simulink model "sl_quadrotorDynamics"  (R2019b)
settings: Solver=VariableStepAuto  StartTime=0.0  StopTime=50  MaxStep=0.1  RelTol=1e-3  EnableMultiTasking=on
InitFcn:
  | % load parameters of the default quadrotor
  | disp('Quadrotor parameters loaded by InitFcn')
  | mdl_quadrotor
values from neighbouring files (symbols this model uses):
  pp_cont =     [sim_parameters.mat]
undefined symbols (not defined in the file or in its folder): quad
libraries: roblocks x1, simulink x1
settings Model: Creator=corkep
settings DataIOCC: LimitDataPoints=on  SaveFormat=Array  ReturnWorkspaceOutputs=off
settings OptimizationCC: BlockReduction=off  BooleanDataType=off  LifeSpan=inf
settings DebuggingCC: SaveWithParameterizedLinksMsg=none  UnderspecifiedInitializationDetection=Classic  MergeDetectMultiDrivingBlocksExec=none  SignalResolutionControl=TryResolveAllWithWarning  SFUnexpectedBacktrackingDiag=warning  SFNoUnconditionalDefaultTransitionDiag=warning  SFExecutionAtInitializationDiag=none  ArithmeticOperatorsInVariantConditions=warning
settings HardwareCC: ProdBitPerPointer=32  ProdBitPerSizeT=32  ProdBitPerPtrDiffT=32  ProdLargestAtomicFloat=None  ProdIntDivRoundTo=Undefined  ProdEndianess=Unspecified  ProdWordSize=32  ProdHWDeviceType=32-bit Generic  TargetUnknown=on
settings ModelReferenceCC: PropagateSignalLabelsOutOfModel=off
settings SFSimCC: SimUseLocalCustomCode=off  CustomCodeUndefinedFunction=UseInterfaceOnly
settings RTWCC: RTWUseLocalCustomCode=off
settings CodeAppCC: StateflowObjectComments=on
settings GRTTargetCC: TargetLangStandard=C89/C90 (ANSI)  GeneratePreprocessorConditionals=Disable all
settings ConfigComp: CovMetricSettings=dw  CovHtmlReporting=on  CovSaveCumulativeToWorkspaceVar=on  CovSaveSingleToWorkspaceVar=on  CovExternalEMLEnable=off  CovSFcnEnable=off

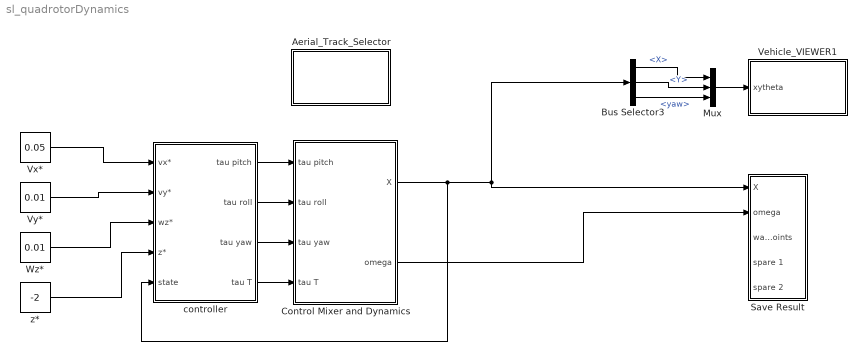
== system sl_quadrotorDynamics ==
  " Save Result" : Subsystem
  Aerial_Track_Selector : Subsystem  mask{the_XL_filename=aerial_robot_waypoints.xlsx, the_racetrack_str=RECT_TRI, the_look_ahead_dist=0.3, the_des_lin_vel=0.1, the_max_ang_vel_deg_sec=60}
      mask prompts: the_XL_filename "EXCEL file (eg: bh.xlsx)"; the_racetrack_str "Racetrack type"; the_look_ahead_dist "Look ahead distance (m)"; the_des_lin_vel "Desired Linear Velocity (m/sec)"; the_max_ang_vel_deg_sec "Max Angular Velocity (deg/sec)"
      mask init:
      | %fprintf('\n ... <%s> and <%s>',the_XL_filename, the_racetrack_str);
      | 
      | A_MASK_OBJ  = Simulink.Mask.get(gcb);
      | A_IMAGE_OBJ = A_MASK_OBJ.getDialogControl('the_track_pic_param');
      | A_IMAGE_OBJ.FilePath = [the_racetrack_str,'.png'];
      | 
      | %--------------------------------------------------------------
      | THE_FILE  = the_XL_filename; 
      | THE_SHEET = the_racetrack_str;
      | my_path_data_T = readtable(THE_FILE, 'Sheet', THE_SHEET);
      | 
      | assignin('base', 'my_path_data_T', my_path_data_T );
      | evalin(  'base', 'pp_cont.Waypoints = [my_path_data_T.X,  my_path_data_T.Y ];' );
      | evalin('base', 'close all');
      | %--------------------------------------------------------------
      | evalin('base', ['pp_cont.LookaheadDistance=',num2str(the_look_ahead_dist),';']);
      | evalin('base', ['pp_cont.DesiredLinearVelocity=',num2str(the_des_lin_vel),';']);
      | evalin('base', ['pp_cont.MaxAngularVelocity=',num2str(the_max_ang_vel_deg_sec*pi/180),';']);
      | %pp_cont.LookaheadDistance     = 0.2;        % m 
      | %pp_cont.DesiredLinearVelocity = 0.1;        % m/s
      | %pp_cont.MaxAngularVelocity    = 60*pi/180;  %radians/second
      mask TypeOptions the_racetrack_str: SPANNER | RECT_TRI | MEDIUM_S_HOME | SMALL_S_HOME | SQUARE | CIRCLE_HOME | L_AND_R_TURNS
      mask DialogControl DescGroupVar Prompt: m_RaceTrack_Selector
      mask DialogControl DescTextVar Prompt: Select the racetrack for your Differential Drive Robot (DDR).  And specify the parameters for your Pure Pursuit controller.
      mask DialogControl Container10 Prompt: RaceTrack
      mask DialogControl Container5 Prompt: PurePursuit
      mask DialogControl Control4 Prompt: If you want some DEFAULT values then click on the button below
      mask DialogControl the_set_def_PP_values Prompt: Set Default values
      mask DialogControl the_set_def_PP_values Callback:
      | set_param(gcb,'the_look_ahead_dist','0.2');
      | set_param(gcb,'the_des_lin_vel','0.1');
      | set_param(gcb,'the_max_ang_vel_deg_sec','60');
      | fprintf('\n *** applied DEFAULT values to PP params ***');
      mask DialogControl Control2 Prompt: As a general rule, the lookahead distance should be larger than the desired linear velocity for a smooth path. The robot might cut corners when the lookahead distance is large. In contrast, a small lookahead distance can result in an unstable path following behavior.
      mask Display: fprintf('%s',the_racetrack_str)
  Bus Selector3 : BusSelector  OutputSignals=X,Y,yaw
  Control Mixer and Dynamics : Subsystem
  Mux : Mux  Inputs=3
  Vehicle_VIEWER1 : Subsystem  mask{wp_mat=pp_cont.Waypoints, veh_ID_num=1, veh_init_xytheta=[0 0 0], Ts=0.1}
      mask prompts: wp_mat "Waypoint matrix for arena [x_col, y_col, z_col, angle_col] (m, deg)"; veh_ID_num "Vehicle ID number"; veh_init_xytheta "Initial pose [x,y, psi]"; Ts "Sample time for updating animation (secs)"
      mask TypeOptions veh_ID_num: 1 | 2 | 3 | 4
      mask DialogControl Control2 Prompt: Animate simulation of Robot
      mask Display: fprintf('veh_ID=%d',veh_ID_num);
  Vx* : Constant  Value=0.05
  Vy* : Constant  Value=0.01
  Wz* : Constant  Value=0.01
  controller : Subsystem
  z* : Constant  Value=-2
  wires:
  Control Mixer and Dynamics/2(omega) -> " Save Result"/2(omega)
  Control Mixer and Dynamics/1(X) -> controller/5(state), Bus Selector3/1, " Save Result"/1(X)
  Bus Selector3/1 -> Mux/1  "<X>"
  Mux/1 -> Vehicle_VIEWER1/1(xytheta)
  Bus Selector3/2 -> Mux/2  "<Y>"
  Bus Selector3/3 -> Mux/3  "<yaw>"
  controller/3(tau yaw) -> Control Mixer and Dynamics/3(tau yaw)
  controller/4(tau T) -> Control Mixer and Dynamics/4(tau T)
  Wz*/1 -> controller/3(wz*)
  z*/1 -> controller/4(z*)
  controller/1(tau pitch) -> Control Mixer and Dynamics/1(tau pitch)
  controller/2(tau roll) -> Control Mixer and Dynamics/2(tau roll)
  Vx*/1 -> controller/1(vx*)
  Vy*/1 -> controller/2(vy*)

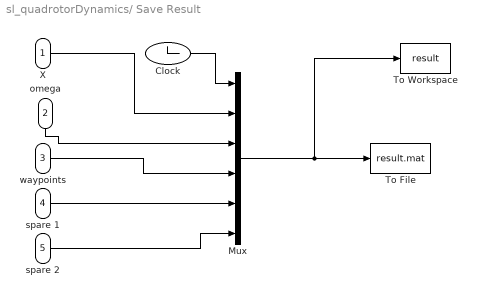
== system sl_quadrotorDynamics/ Save Result ==
  X : Inport
  omega : Inport  Port=2
  waypoints : Inport  Port=3
  spare 1 : Inport  Port=4
  spare 2 : Inport  Port=5
  Clock : Clock
  Mux : Mux  Inputs=6
  To File : ToFile  Filename=result.mat  MatrixName=result  SaveFormat=Timeseries
  To Workspace : ToWorkspace  VariableName=result  SampleTime=-1
  wires:
  Clock/1 -> Mux/1
  omega/1 -> Mux/3
  Mux/1 -> To Workspace/1, To File/1
  X/1 -> Mux/2
  spare 1/1 -> Mux/5
  spare 2/1 -> Mux/6
  waypoints/1 -> Mux/4

== system sl_quadrotorDynamics/Aerial_Track_Selector ==

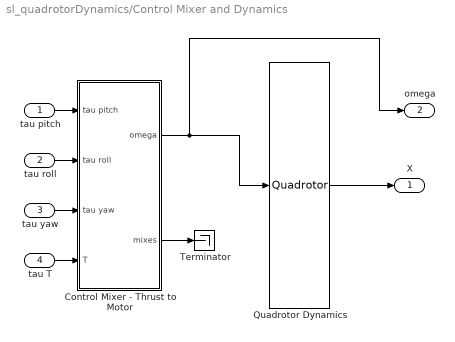
== system sl_quadrotorDynamics/Control Mixer and Dynamics ==
  tau pitch : Inport
  tau roll : Inport  Port=2
  tau yaw : Inport  Port=3
  tau T : Inport  Port=4
  Control Mixer - Thrust to Motor : Subsystem
  Quadrotor Dynamics : roblocks/Dynamics/Quadrotor  quad=quad
      link override Dynamics: FunctionName=nrotor_dynamics
  Terminator : Terminator
  X : Outport  VectorParamsAs1DForOutWhenUnconnected=off
  omega : Outport  Port=2  VectorParamsAs1DForOutWhenUnconnected=off
  wires:
  Quadrotor Dynamics/1 -> X/1
  Control Mixer - Thrust to Motor/2(mixes) -> Terminator/1
  tau pitch/1 -> Control Mixer - Thrust to Motor/1(tau pitch)
  tau roll/1 -> Control Mixer - Thrust to Motor/2(tau roll)
  tau yaw/1 -> Control Mixer - Thrust to Motor/3(tau yaw)
  tau T/1 -> Control Mixer - Thrust to Motor/4(T)
  Control Mixer - Thrust to Motor/1(omega) -> Quadrotor Dynamics/1, omega/1

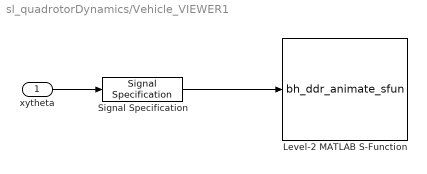
== system sl_quadrotorDynamics/Vehicle_VIEWER1 ==
  xytheta : Inport
  Level-2 MATLAB S-Function : M-S-Function  FunctionName=bh_ddr_animate_sfun  Parameters=Ts, wp_mat, veh_ID_num, veh_init_xytheta
  Signal Specification : SignalSpecification  Dimensions=3
  wires:
  xytheta/1 -> Signal Specification/1
  Signal Specification/1 -> Level-2 MATLAB S-Function/1

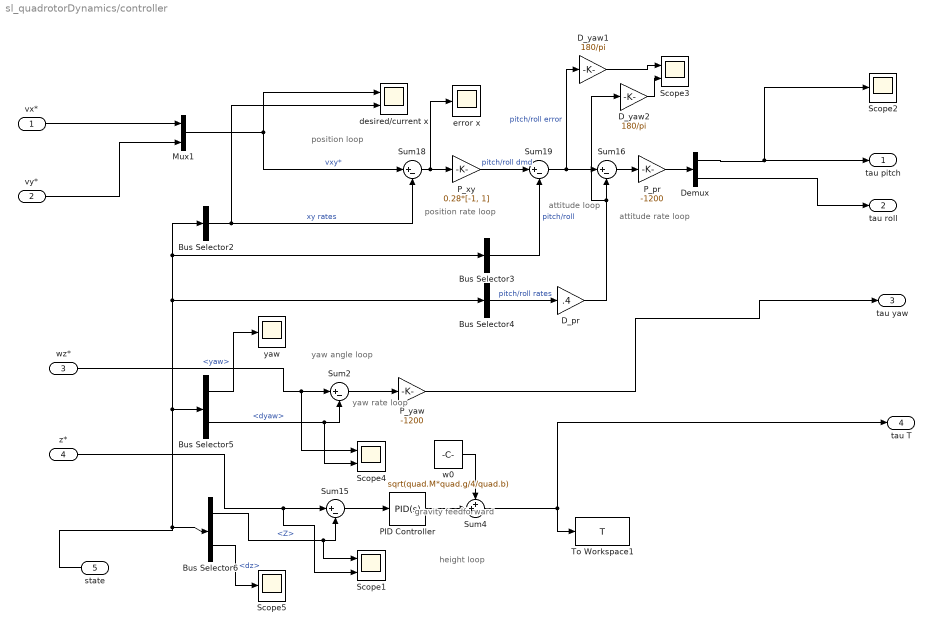
== system sl_quadrotorDynamics/controller ==
  note: gravity feedforward
  note: attitude rate
      | loop
  note: attitude
      | loop
  note: position rate
      | loop
  note: position
      | loop
  note: yaw rate
      | loop
  note: yaw angle
      | loop
  note: height
      | loop
  vx* : Inport
  vy* : Inport  Port=2
  wz* : Inport  Port=3
  z* : Inport  Port=4
  state : Inport  Port=5
  Bus Selector2 : BusSelector  OutputSignals=dx,dy  OutputAsBus=on
  Bus Selector3 : BusSelector  OutputSignals=pitch,roll  OutputAsBus=on
  Bus Selector4 : BusSelector  OutputSignals=dpitch,droll  OutputAsBus=on
  Bus Selector5 : BusSelector  OutputSignals=yaw,dyaw
  Bus Selector6 : BusSelector  OutputSignals=Z,dz
  D_pr : Gain  Gain=.4
  D_yaw1 : Gain  Gain=180/pi
  D_yaw2 : Gain  Gain=180/pi
  Demux : Demux  Outputs=2
  Mux1 : Mux  Inputs=2
  PID Controller : simulink/Continuous/PID Controller  Controller=PID  Form=Parallel  TimeDomain=Continuous-time  SampleTime=-1  IntegratorMethod=Forward Euler  FilterMethod=Forward Euler  ControllerParametersSource=internal  P=-8.79853091186098  I=-0.449865753789399  D=-42.04549910981  UseFilter=on  N=5.45397025421619  TunerSelectOption=Transfer Function Based (PID Tuner App)  InitialConditionSource=internal  InitialConditionForIntegrator=0  InitialConditionForFilter=0  DifferentiatorICPrevScaledInput=0  ExternalReset=none  TrackingMode=off  Kt=1  LimitOutput=off  UpperSaturationLimit=inf  LowerSaturationLimit=-inf  LinearizeAsGain=on  AntiWindupMode=none  Kb=1  POutMin=[]  POutMax=[]  IOutMin=[]  IOutMax=[]  DOutMin=[]  DOutMax=[]  NOutMin=[]  NOutMax=[]  SumOutMin=[]  SumOutMax=[]  SaturationOutMin=[]  SaturationOutMax=[]  PParamMin=[]  PParamMax=[]  IParamMin=[]  IParamMax=[]  DParamMin=[]  DParamMax=[]  NParamMin=[]  NParamMax=[]  KbParamMin=[]  KbParamMax=[]  KtParamMin=[]  KtParamMax=[]  KbOutMin=[]  KbOutMax=[]  KtOutMin=[]  KtOutMax=[]  IntegratorOutMin=[]  IntegratorOutMax=[]  FilterOutMin=[]  FilterOutMax=[]  SumI1OutMin=[]  SumI1OutMax=[]  SumI2OutMin=[]  SumI2OutMax=[]  SumI3OutMin=[]  SumI3OutMax=[]  SumI4OutMin=[]  SumI4OutMax=[]  SumDOutMin=[]  SumDOutMax=[]  DifferentiatorOutMin=[]  DifferentiatorOutMax=[]  FilterDiffOutCoefMin=[]  FilterDiffOutCoefMax=[]  ReciprocalOutMin=[]  ReciprocalOutMax=[]  SumDenOutMin=[]  SumDenOutMax=[]  SumNumOutMin=[]  SumNumOutMax=[]  DivideOutMin=[]  DivideOutMax=[]  IntegratorContinuousStateAttributes=''  IntegratorStateMustResolveToSignalObject=off  IntegratorRTWStateStorageClass=Auto  FilterContinuousStateAttributes=''  FilterStateMustResolveToSignalObject=off  FilterRTWStateStorageClass=Auto  ParallelPVariant=InternalParameters  IdealPVariant=Disabled  IVariant=InternalParameters  DVariant=InternalParameters  IntegratorVariant=Continuous  SatVariant=Disabled  AWVariant=Passthrough  PCopyVariant=Disabled  TRVariant=Disabled  FdbkBlocksVariant=Forward  IdealPFdbkVariant=Disabled  SatFdbkVariant=Disabled  DerivativeFilterVariant=ContFilter  NVariant=InternalParameters  NCopyVariant=Disabled  FilterICVariant=InternalICsFilter  IntegratorICVariant=InternalICs  ExternalResetVariant=Disabled  TRSumVariant=Passthrough  SumFdbkVariant=Disabled  SumVariant=Sum_PID
  P_pr : Gain  Gain=-1200
  P_xy : Gain  Gain=0.28*[-1, 1]
  P_yaw : Gain  Gain=-1200
  Scope1 : Scope  NumInputPorts=2
  Scope2 : Scope
  Scope3 : Scope  NumInputPorts=2
  Scope4 : Scope  NumInputPorts=2
  Scope5 : Scope
  Sum{2,15..16,18..19} (5 alike) : Sum  Inputs=|+-
  Sum4 : Sum  Inputs=++|
  To Workspace1 : ToWorkspace  VariableName=T  SampleTime=-1
  desired/current x : Scope  NumInputPorts=2
  error x : Scope
  w0 : Constant  Value=sqrt(quad.M*quad.g/4/quad.b)  SampleTime=0
  yaw : Scope
  tau pitch : Outport
  tau roll : Outport  Port=2
  tau yaw : Outport  Port=3
  tau T : Outport  Port=4
  wires:
  PID Controller/1 -> Sum4/2
  D_yaw1/1 -> Scope3/1
  Bus Selector2/1 -> Sum18/2, desired/current x/2  "xy rates"
  vy*/1 -> Mux1/2
  P_yaw/1 -> tau yaw/1
  Demux/1 -> tau pitch/1, Scope2/1
  P_pr/1 -> Demux/1
  w0/1 -> Sum4/1
  Sum18/1 -> error x/1, P_xy/1
  Sum15/1 -> PID Controller/1
  D_pr/1 -> D_yaw2/1, Sum16/2
  Sum19/1 -> D_yaw1/1, Sum16/1  "pitch/roll error"
  Mux1/1 -> Sum18/1, desired/current x/1  "vxy*"
  Bus Selector5/2 -> Sum2/2, Scope4/2  "<dyaw>"
  Sum4/1 -> To Workspace1/1, tau T/1
  Demux/2 -> tau roll/1
  wz*/1 -> Scope4/1, Sum2/1
  Bus Selector3/1 -> Sum19/2  "pitch/roll"
  Sum2/1 -> P_yaw/1
  Sum16/1 -> P_pr/1
  state/1 -> Bus Selector4/1, Bus Selector3/1, Bus Selector2/1, Bus Selector5/1, Bus Selector6/1
  P_xy/1 -> Sum19/1  "pitch/roll dmd"
  Bus Selector4/1 -> D_pr/1  "pitch/roll rates"
  vx*/1 -> Mux1/1
  z*/1 -> Scope1/2, Sum15/1
  D_yaw2/1 -> Scope3/2
  Bus Selector6/1 -> Scope1/1, Sum15/2  "<Z>"
  Bus Selector6/2 -> Scope5/1  "<dz>"
  Bus Selector5/1 -> yaw/1  "<yaw>"

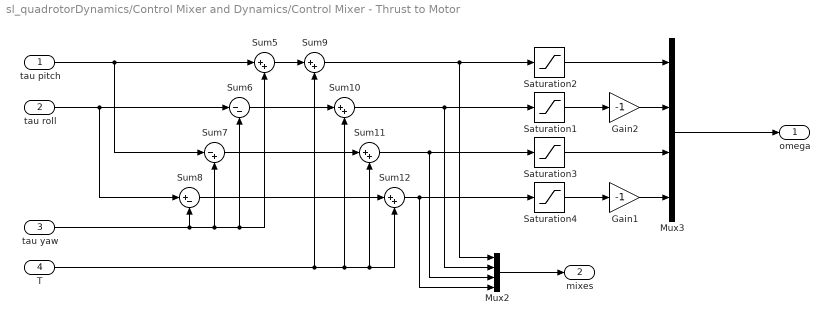
== system sl_quadrotorDynamics/Control Mixer and Dynamics/Control Mixer - Thrust to Motor ==
  tau pitch : Inport
  tau roll : Inport  Port=2
  tau yaw : Inport  Port=3
  T : Inport  Port=4
  Gain1 : Gain  Gain=-1
  Gain2 : Gain  Gain=-1
  Mux2 : Mux
  Mux3 : Mux
  Saturation{1..4} (4 alike) : Saturate  UpperLimit=1000  LowerLimit=700
  Sum{5,9..12} (5 alike) : Sum  Inputs=|++  SaturateOnIntegerOverflow=on  InputSameDT=on  OutDataTypeStr=Inherit: Same as first input
  Sum6 : Sum  Inputs=|--  SaturateOnIntegerOverflow=on  InputSameDT=on  OutDataTypeStr=Inherit: Same as first input
  Sum7 : Sum  Inputs=|-+  SaturateOnIntegerOverflow=on  InputSameDT=on  OutDataTypeStr=Inherit: Same as first input
  Sum8 : Sum  Inputs=|+-  SaturateOnIntegerOverflow=on  InputSameDT=on  OutDataTypeStr=Inherit: Same as first input
  omega : Outport  VectorParamsAs1DForOutWhenUnconnected=off
  mixes : Outport  Port=2  VectorParamsAs1DForOutWhenUnconnected=off
  wires:
  Sum7/1 -> Sum11/1
  tau roll/1 -> Sum6/1, Sum8/1
  Mux2/1 -> mixes/1
  Gain2/1 -> Mux3/2
  Sum8/1 -> Sum12/1
  Sum6/1 -> Sum10/1
  tau pitch/1 -> Sum5/1, Sum7/1
  Mux3/1 -> omega/1
  Sum10/1 -> Saturation1/1, Mux2/2
  Sum12/1 -> Saturation4/1, Mux2/4
  Saturation1/1 -> Gain2/1
  Saturation3/1 -> Mux3/3
  T/1 -> Sum11/2, Sum12/2, Sum10/2, Sum9/2
  tau yaw/1 -> Sum8/2, Sum7/2, Sum6/2, Sum5/2
  Saturation4/1 -> Gain1/1
  Sum9/1 -> Saturation2/1, Mux2/1
  Sum11/1 -> Saturation3/1, Mux2/3
  Saturation2/1 -> Mux3/1
  Sum5/1 -> Sum9/1
  Gain1/1 -> Mux3/4
